simulink model "gas_pedal"  (R2014b)
settings: Solver=ode45  StartTime=0.0  StopTime=10.0  RelTol=1e-3
undefined symbols (not defined in the file or in its folder): AirStep, tau_th
settings Model: Creator=Niclas  LastModifiedBy=danfa688

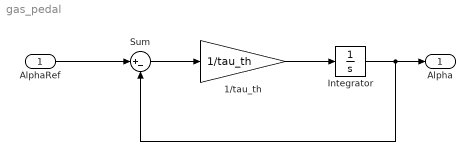
== system gas_pedal ==
  AlphaRef : Inport
  1/tau_th : Gain  Gain=1/tau_th  SaturateOnIntegerOverflow=on  OutDataTypeStr=Inherit: Same as input  ParamDataTypeStr=Inherit: Same as input
  Integrator : Integrator  InitialCondition=AirStep.alpha_ref(1)
  Sum : Sum  Inputs=|+-  SaturateOnIntegerOverflow=on
  Alpha : Outport
  wires:
  AlphaRef/1 -> Sum/1
  Sum/1 -> 1/tau_th/1
  Integrator/1 -> Alpha/1, Sum/2
  1/tau_th/1 -> Integrator/1
